simulink model "simple_arda_mpc_tune_me"  (R2021b)
settings: Solver=VariableStepAuto  StartTime=0  StopTime=10000  FixedStep=0.1  RelTol=1e-3
PreLoadFcn:
  | % Setup model parameters
  |                 % Sample time
  |                 %Ts = 0.1;
  |                 % Simulation stop time ("TimeOut")
  |                 %stop_time = 8000;
  |                 % Temperature
  |                 %T_init = 20 + 273.1755;
  |                % T_final = 294.1755;
  |               %  T_env = 20 + 273.15; %#ok<*NASGU>
  |              %   % Heater
  |                 %u_volts_heater_init = 0; % volts
  |                 % Pressure
  |                 %p_init = 101.325; % kPa
  |                 %p_env = 101.325; % kPa
  |                 % Relative humidity and steam
  |                 %phi_init = 0.4987;
  |                 %phi_final = 0.6;
  |                 %phi_env = 0.1;
  |                 %u_steam_init = 0;
  |                 %T_steam = 130 + 273.15;
  |                 % Volumetric flow rate
  |                 %u_volts_fan_init = 1;
  |                 %flow_init = 5.8e-3;
  |                 %flow_final = 0.18;
  |                 % Smooth ramp input parameters
  |                 %smooth_step_heater = make_smooth_step(0, T_init, T_final, Ts, stop_time, 'T_g');
  |                 %smooth_step_steam = make_smooth_step(0, phi_init, phi_final, Ts, stop_time, 'phi');
  |                 %smooth_step_fan = make_smooth_step(0, flow_init, flow_final, Ts, stop_time, 'flow');
  |                 % Parameters to vary for linearization
  |                 % Pipes
  |                 %pipe_length1 = 1; % meters
  |                 %pipe_length2 = 1;
  |                 %pipe_length3 = 1;
  |                 %pipe_cross_sectional_area1 = pi*(2*2.54/2)^2; % cm^2
  |                 %pipe_cross_sectional_area2 = pi*(2*2.54/2)^2;
  |                 %pipe_cross_sectional_area3 = pi*(2*2.54/2)^2;
  |                 %pipe_hydraulic_diameter1 = 2*2.54; %cm
  |                 %pipe_hydraulic_diameter2 = 2*2.54; %cm
  |                 %pipe_hydraulic_diameter3 = 2*2.54; %cm
  |                 % Thermal masses
  |                 %thermal_mass1 = 1; % kg
  |                 %thermal_mass2 = 1; % kg
  |                 %thermal_mass3 = 1; % kg
  |                 %thermal_mass4 = 1; % kg
  |                 %thermal_mass5 = 1; % kg
  |                 %specific_heat1 = 447; % J/(K*kg)
  |                 %specific_heat2 = 447; % J/(K*kg)
  |                 %specific_heat3 = 447; % J/(K*kg)
  |                 %specific_heat4 = 447; % J/(K*kg)
  |                 %specific_heat5 = 447; % J/(K*kg)
InitFcn:
  | load('bob.mat')
model workspace (MAT data in the model file):
  simple_arda_mpc_tune_me_sdosession = sldodialogs.data.SessionData
  simple_arda_mpc_tune_me_sdosession.Version = '3.0'
  simple_arda_mpc_tune_me_sdosession.Data.ModelName = 'simple_arda_mpc_tune_me'
  simple_arda_mpc_tune_me_sdosession.Data.ToolType = 'ResponseOptimization'
  simple_arda_mpc_tune_me_sdosession.Data.GUIOptions.NoPromptClose = 0
  simple_arda_mpc_tune_me_sdosession.Data.Workspace.LocalWorkspace.BlockReq = sldodialogs.databrowser.BlockRequirementData
  simple_arda_mpc_tune_me_sdosession.Data.Workspace.LocalWorkspace.BlockReq.Name = 'BlockReq'
  simple_arda_mpc_tune_me_sdosession.Data.Workspace.LocalWorkspace.BlockReq.Block = 'simple_arda_mpc_tune_me/check_T'
  simple_arda_mpc_tune_me_sdosession.Data.Workspace.LocalWorkspace.BlockReq_1 = sldodialogs.databrowser.BlockRequirementData
  simple_arda_mpc_tune_me_sdosession.Data.Workspace.LocalWorkspace.BlockReq_1.Name = 'BlockReq_1'
  simple_arda_mpc_tune_me_sdosession.Data.Workspace.LocalWorkspace.BlockReq_1.Block = 'simple_arda_mpc_tune_me/check_flow'
  simple_arda_mpc_tune_me_sdosession.Data.Workspace.LocalWorkspace.BlockReq_2 = sldodialogs.databrowser.BlockRequirementData
  simple_arda_mpc_tune_me_sdosession.Data.Workspace.LocalWorkspace.BlockReq_2.Name = 'BlockReq_2'
  simple_arda_mpc_tune_me_sdosession.Data.Workspace.LocalWorkspace.BlockReq_2.Block = 'simple_arda_mpc_tune_me/check_phi'
  simple_arda_mpc_tune_me_sdosession.Data.Workspace.LocalWorkspace.DesignVars(1) = param.Continuous
  simple_arda_mpc_tune_me_sdosession.Data.Workspace.LocalWorkspace.DesignVars(1).Minimum_ = 0
  simple_arda_mpc_tune_me_sdosession.Data.Workspace.LocalWorkspace.DesignVars(1).Maximum_ = 4
  simple_arda_mpc_tune_me_sdosession.Data.Workspace.LocalWorkspace.DesignVars(1).Scale_ = 2
  simple_arda_mpc_tune_me_sdosession.Data.Workspace.LocalWorkspace.DesignVars(1).Size_ = [1 1]
  simple_arda_mpc_tune_me_sdosession.Data.Workspace.LocalWorkspace.DesignVars(1).Value_ = 1.99942074063
  simple_arda_mpc_tune_me_sdosession.Data.Workspace.LocalWorkspace.DesignVars(1).pID = paramid.Variable
  simple_arda_mpc_tune_me_sdosession.Data.Workspace.LocalWorkspace.DesignVars(1).pID.Name = 'u1_wt'
  simple_arda_mpc_tune_me_sdosession.Data.Workspace.LocalWorkspace.DesignVars(2) = param.Continuous
  simple_arda_mpc_tune_me_sdosession.Data.Workspace.LocalWorkspace.DesignVars(2).Minimum_ = 3
  simple_arda_mpc_tune_me_sdosession.Data.Workspace.LocalWorkspace.DesignVars(2).Maximum_ = 6
  simple_arda_mpc_tune_me_sdosession.Data.Workspace.LocalWorkspace.DesignVars(2).Scale_ = 8
  simple_arda_mpc_tune_me_sdosession.Data.Workspace.LocalWorkspace.DesignVars(2).Size_ = [1 1]
  simple_arda_mpc_tune_me_sdosession.Data.Workspace.LocalWorkspace.DesignVars(2).Value_ = 4.47918835767
  simple_arda_mpc_tune_me_sdosession.Data.Workspace.LocalWorkspace.DesignVars(2).pID = paramid.Variable
  simple_arda_mpc_tune_me_sdosession.Data.Workspace.LocalWorkspace.DesignVars(2).pID.Name = 'u2_wt'
  simple_arda_mpc_tune_me_sdosession.Data.Workspace.LocalWorkspace.DesignVars(3) = param.Continuous
  simple_arda_mpc_tune_me_sdosession.Data.Workspace.LocalWorkspace.DesignVars(3).Minimum_ = 6
  simple_arda_mpc_tune_me_sdosession.Data.Workspace.LocalWorkspace.DesignVars(3).Maximum_ = 10
  simple_arda_mpc_tune_me_sdosession.Data.Workspace.LocalWorkspace.DesignVars(3).Scale_ = 8
  simple_arda_mpc_tune_me_sdosession.Data.Workspace.LocalWorkspace.DesignVars(3).Size_ = [1 1]
  simple_arda_mpc_tune_me_sdosession.Data.Workspace.LocalWorkspace.DesignVars(3).Value_ = 6
  simple_arda_mpc_tune_me_sdosession.Data.Workspace.LocalWorkspace.DesignVars(3).pID = paramid.Variable
  simple_arda_mpc_tune_me_sdosession.Data.Workspace.LocalWorkspace.DesignVars(3).pID.Name = 'u3_wt'
  simple_arda_mpc_tune_me_sdosession.Data.Workspace.LocalWorkspace.DesignVars(4) = param.Continuous
  simple_arda_mpc_tune_me_sdosession.Data.Workspace.LocalWorkspace.DesignVars(4).Minimum_ = 850
  simple_arda_mpc_tune_me_sdosession.Data.Workspace.LocalWorkspace.DesignVars(4).Maximum_ = 1050
  simple_arda_mpc_tune_me_sdosession.Data.Workspace.LocalWorkspace.DesignVars(4).Scale_ = 1024
  simple_arda_mpc_tune_me_sdosession.Data.Workspace.LocalWorkspace.DesignVars(4).Size_ = [1 1]
  simple_arda_mpc_tune_me_sdosession.Data.Workspace.LocalWorkspace.DesignVars(4).Value_ = 1050
  simple_arda_mpc_tune_me_sdosession.Data.Workspace.LocalWorkspace.DesignVars(4).pID = paramid.Variable
  simple_arda_mpc_tune_me_sdosession.Data.Workspace.LocalWorkspace.DesignVars(4).pID.Name = 'y1_wt'
  simple_arda_mpc_tune_me_sdosession.Data.Workspace.LocalWorkspace.DesignVars(5) = param.Continuous
  simple_arda_mpc_tune_me_sdosession.Data.Workspace.LocalWorkspace.DesignVars(5).Minimum_ = 38
  simple_arda_mpc_tune_me_sdosession.Data.Workspace.LocalWorkspace.DesignVars(5).Maximum_ = 46
  simple_arda_mpc_tune_me_sdosession.Data.Workspace.LocalWorkspace.DesignVars(5).Scale_ = 64
  simple_arda_mpc_tune_me_sdosession.Data.Workspace.LocalWorkspace.DesignVars(5).Size_ = [1 1]
  simple_arda_mpc_tune_me_sdosession.Data.Workspace.LocalWorkspace.DesignVars(5).Value_ = 46
  simple_arda_mpc_tune_me_sdosession.Data.Workspace.LocalWorkspace.DesignVars(5).pID = paramid.Variable
  simple_arda_mpc_tune_me_sdosession.Data.Workspace.LocalWorkspace.DesignVars(5).pID.Name = 'y2_wt'
  simple_arda_mpc_tune_me_sdosession.Data.Workspace.LocalWorkspace.DesignVars(6) = param.Continuous
  simple_arda_mpc_tune_me_sdosession.Data.Workspace.LocalWorkspace.DesignVars(6).Minimum_ = 200
  simple_arda_mpc_tune_me_sdosession.Data.Workspace.LocalWorkspace.DesignVars(6).Maximum_ = 250
  simple_arda_mpc_tune_me_sdosession.Data.Workspace.LocalWorkspace.DesignVars(6).Scale_ = 256
  simple_arda_mpc_tune_me_sdosession.Data.Workspace.LocalWorkspace.DesignVars(6).Size_ = [1 1]
  simple_arda_mpc_tune_me_sdosession.Data.Workspace.LocalWorkspace.DesignVars(6).Value_ = 200
  simple_arda_mpc_tune_me_sdosession.Data.Workspace.LocalWorkspace.DesignVars(6).pID = paramid.Variable
  simple_arda_mpc_tune_me_sdosession.Data.Workspace.LocalWorkspace.DesignVars(6).pID.Name = 'y3_wt'
  simple_arda_mpc_tune_me_sdosession.Data.Workspace.LocalWorkspace.DesignVars(7) = param.Continuous
  simple_arda_mpc_tune_me_sdosession.Data.Workspace.LocalWorkspace.DesignVars(7).Minimum_ = 4000
  simple_arda_mpc_tune_me_sdosession.Data.Workspace.LocalWorkspace.DesignVars(7).Maximum_ = 6000
  simple_arda_mpc_tune_me_sdosession.Data.Workspace.LocalWorkspace.DesignVars(7).Scale_ = 8192
  simple_arda_mpc_tune_me_sdosession.Data.Workspace.LocalWorkspace.DesignVars(7).Size_ = [1 1]
  simple_arda_mpc_tune_me_sdosession.Data.Workspace.LocalWorkspace.DesignVars(7).Value_ = 5000
  simple_arda_mpc_tune_me_sdosession.Data.Workspace.LocalWorkspace.DesignVars(7).pID = paramid.Variable
  simple_arda_mpc_tune_me_sdosession.Data.Workspace.LocalWorkspace.DesignVars(7).pID.Name = 'u1p_wt'
  simple_arda_mpc_tune_me_sdosession.Data.Workspace.LocalWorkspace.DesignVars(8) = param.Continuous
  simple_arda_mpc_tune_me_sdosession.Data.Workspace.LocalWorkspace.DesignVars(8).Minimum_ = 2000
  simple_arda_mpc_tune_me_sdosession.Data.Workspace.LocalWorkspace.DesignVars(8).Maximum_ = 4000
  simple_arda_mpc_tune_me_sdosession.Data.Workspace.LocalWorkspace.DesignVars(8).Scale_ = 4096
  simple_arda_mpc_tune_me_sdosession.Data.Workspace.LocalWorkspace.DesignVars(8).Size_ = [1 1]
  simple_arda_mpc_tune_me_sdosession.Data.Workspace.LocalWorkspace.DesignVars(8).Value_ = 3000
  simple_arda_mpc_tune_me_sdosession.Data.Workspace.LocalWorkspace.DesignVars(8).pID = paramid.Variable
  simple_arda_mpc_tune_me_sdosession.Data.Workspace.LocalWorkspace.DesignVars(8).pID.Name = 'u2p_wt'
  simple_arda_mpc_tune_me_sdosession.Data.Workspace.LocalWorkspace.DesignVars(9) = param.Continuous
  simple_arda_mpc_tune_me_sdosession.Data.Workspace.LocalWorkspace.DesignVars(9).Minimum_ = 1000
  simple_arda_mpc_tune_me_sdosession.Data.Workspace.LocalWorkspace.DesignVars(9).Maximum_ = 3000
  simple_arda_mpc_tune_me_sdosession.Data.Workspace.LocalWorkspace.DesignVars(9).Scale_ = 2048
  simple_arda_mpc_tune_me_sdosession.Data.Workspace.LocalWorkspace.DesignVars(9).Size_ = [1 1]
  simple_arda_mpc_tune_me_sdosession.Data.Workspace.LocalWorkspace.DesignVars(9).Value_ = 2000
  simple_arda_mpc_tune_me_sdosession.Data.Workspace.LocalWorkspace.DesignVars(9).pID = paramid.Variable
  simple_arda_mpc_tune_me_sdosession.Data.Workspace.LocalWorkspace.DesignVars(9).pID.Name = 'u3p_wt'
  simple_arda_mpc_tune_me_sdosession.Data.Workspace.LocalWorkspace.DesignVars(10) = param.Continuous
  simple_arda_mpc_tune_me_sdosession.Data.Workspace.LocalWorkspace.DesignVars(10).Minimum_ = 1
  simple_arda_mpc_tune_me_sdosession.Data.Workspace.LocalWorkspace.DesignVars(10).Maximum_ = 4
  simple_arda_mpc_tune_me_sdosession.Data.Workspace.LocalWorkspace.DesignVars(10).Scale_ = 8
  simple_arda_mpc_tune_me_sdosession.Data.Workspace.LocalWorkspace.DesignVars(10).Size_ = [1 1]
  simple_arda_mpc_tune_me_sdosession.Data.Workspace.LocalWorkspace.DesignVars(10).Value_ = 5
  simple_arda_mpc_tune_me_sdosession.Data.Workspace.LocalWorkspace.DesignVars(10).pID = paramid.Variable
  simple_arda_mpc_tune_me_sdosession.Data.Workspace.LocalWorkspace.DesignVars(10).pID.Name = 'control_horizon'
  simple_arda_mpc_tune_me_sdosession.Data.Workspace.LocalWorkspace.DesignVars(11) = param.Continuous
  simple_arda_mpc_tune_me_sdosession.Data.Workspace.LocalWorkspace.DesignVars(11).Minimum_ = 5
  simple_arda_mpc_tune_me_sdosession.Data.Workspace.LocalWorkspace.DesignVars(11).Maximum_ = 10
  simple_arda_mpc_tune_me_sdosession.Data.Workspace.LocalWorkspace.DesignVars(11).Scale_ = 16
  simple_arda_mpc_tune_me_sdosession.Data.Workspace.LocalWorkspace.DesignVars(11).Size_ = [1 1]
  simple_arda_mpc_tune_me_sdosession.Data.Workspace.LocalWorkspace.DesignVars(11).Value_ = 10
  simple_arda_mpc_tune_me_sdosession.Data.Workspace.LocalWorkspace.DesignVars(11).pID = paramid.Variable
  simple_arda_mpc_tune_me_sdosession.Data.Workspace.LocalWorkspace.DesignVars(11).pID.Name = 'prediction_horizon'
  simple_arda_mpc_tune_me_sdosession.Data.Workspace.LocalWorkspace.ReqValues(1).Name = 'simple_arda_mpc_tune_me/check_T (Upper)'
  simple_arda_mpc_tune_me_sdosession.Data.Workspace.LocalWorkspace.ReqValues(1).Type = '<='
  simple_arda_mpc_tune_me_sdosession.Data.Workspace.LocalWorkspace.ReqValues(1).Value = [-0.0594490574926; -0.054838686924; -0.0546633029945; -0.000573871237779; 0.0439457003428; 0.0538224147144; 0.0538106463197; 436.002710593]
  simple_arda_mpc_tune_me_sdosession.Data.Workspace.LocalWorkspace.ReqValues(1).DisplayValue = [-0.0594490574926; -0.054838686924; -0.0546633029945; -0.000573871237779; 0.0439457003428; 0.0538224147144; 0.0538106463197; 436.002710593]
  simple_arda_mpc_tune_me_sdosession.Data.Workspace.LocalWorkspace.ReqValues(2).Name = 'simple_arda_mpc_tune_me/check_flow (Upper)'
  simple_arda_mpc_tune_me_sdosession.Data.Workspace.LocalWorkspace.ReqValues(2).Type = '<='
  simple_arda_mpc_tune_me_sdosession.Data.Workspace.LocalWorkspace.ReqValues(2).Value = [-0.954656561585; -0.967742763883; -0.947580933078; -1.05584644778; 0.959275239402; 0.975371838836; 0.991305602274; 924.477313265]
  simple_arda_mpc_tune_me_sdosession.Data.Workspace.LocalWorkspace.ReqValues(2).DisplayValue = [-0.954656561585; -0.967742763883; -0.947580933078; -1.05584644778; 0.959275239402; 0.975371838836; 0.991305602274; 924.477313265]
  simple_arda_mpc_tune_me_sdosession.Data.Workspace.LocalWorkspace.ReqValues(3).Name = 'simple_arda_mpc_tune_me/check_phi (Upper)'
  simple_arda_mpc_tune_me_sdosession.Data.Workspace.LocalWorkspace.ReqValues(3).Type = '<='
  simple_arda_mpc_tune_me_sdosession.Data.Workspace.LocalWorkspace.ReqValues(3).Value = [-0.400637667521; 0.0893932441366]
  simple_arda_mpc_tune_me_sdosession.Data.Workspace.LocalWorkspace.ReqValues(3).DisplayValue = [-0.400637667521; 0.0893932441366]
  simple_arda_mpc_tune_me_sdosession.Data.Workspace.LocalWorkspace.ReqValues(4).Name = 'simple_arda_mpc_tune_me/check_phi (Lower)'
  simple_arda_mpc_tune_me_sdosession.Data.Workspace.LocalWorkspace.ReqValues(4).Type = '>='
  simple_arda_mpc_tune_me_sdosession.Data.Workspace.LocalWorkspace.ReqValues(4).Value = [-0.599166284275; -0.330396343818]
  simple_arda_mpc_tune_me_sdosession.Data.Workspace.LocalWorkspace.ReqValues(4).DisplayValue = [0.599166284275; 0.330396343818]
  simple_arda_mpc_tune_me_sdosession.Data.Workspace.HiddenWorkspace = []
  simple_arda_mpc_tune_me_sdosession.Data.ToolData.PlotManager.Plots(1).Class = 'block'
  simple_arda_mpc_tune_me_sdosession.Data.ToolData.PlotManager.Plots(1).Sources = {'simple_arda_mpc_tune_me/check_T'}
  simple_arda_mpc_tune_me_sdosession.Data.ToolData.PlotManager.Plots(2).Class = 'block'
  simple_arda_mpc_tune_me_sdosession.Data.ToolData.PlotManager.Plots(2).Sources = {'simple_arda_mpc_tune_me/check_flow'}
  simple_arda_mpc_tune_me_sdosession.Data.ToolData.PlotManager.Plots(3).Class = 'block'
  simple_arda_mpc_tune_me_sdosession.Data.ToolData.PlotManager.Plots(3).Sources = {'simple_arda_mpc_tune_me/check_phi'}
  simple_arda_mpc_tune_me_sdosession.Data.ToolData.PlotManager.Plots(4).Class = 'sldoplots.IterPlot'
  simple_arda_mpc_tune_me_sdosession.Data.ToolData.PlotManager.Plots(4).Sources = {'DesignVars'}
  simple_arda_mpc_tune_me_sdosession.Data.ToolData.PlotManager.Tiling : java.lang.String (value not decoded)
  simple_arda_mpc_tune_me_sdosession.Data.ToolData.DialogManager = []
  simple_arda_mpc_tune_me_sdosession.Data.ToolData.ResponseOptimization.Options = sdo.OptimizeOptions
  simple_arda_mpc_tune_me_sdosession.Data.ToolData.ResponseOptimization.Options.Restarts = 2
  simple_arda_mpc_tune_me_sdosession.Data.ToolData.ResponseOptimization.Options.UseParallel = 1
  simple_arda_mpc_tune_me_sdosession.Data.ToolData.ResponseOptimization.Options.ParallelFileDependencies = {'C:/Users/dmeissner/stuff/arda/work/integration/bob.mat'; 'C:/Users/dmeissner/stuff/arda/work/integration/data_dictionary1.sldd'; 'C:/Users/dmeissner/stuff/arda/work/integration/plant.slx'; 'C:/Users/dmeissner/stuff/arda/work/integration/simple_arda_mpc_tune_me.slx'; 'C:/Users/dmeissner/stuff/arda/work/integration/simple_arda_mpc_tune_me.slxc'}
  simple_arda_mpc_tune_me_sdosession.Data.ToolData.ResponseOptimization.Options.OptimizedModel = 'simple_arda_mpc_tune_me'
  simple_arda_mpc_tune_me_sdosession.Data.ToolData.ResponseOptimization.Options.Version = 2
  simple_arda_mpc_tune_me_sdosession.Data.ToolData.ResponseOptimization.GUIOptions.ModelTimeOut = 15000
  simple_arda_mpc_tune_me_sdosession.Data.ToolData.ResponseOptimization.GUIOptions.ComputeOperatingPoint = 0
  simple_arda_mpc_tune_me_sdosession.Data.ToolData.ResponseOptimization.GUIOptions.ShowProgress = 1
  simple_arda_mpc_tune_me_sdosession.Data.ToolData.ResponseOptimization.GUIOptions.ShowParamTrajectory = 1
  simple_arda_mpc_tune_me_sdosession.Data.ToolData.ResponseOptimization.GUIOptions.UpdatePlots = 0
  simple_arda_mpc_tune_me_sdosession.Data.ToolData.ResponseOptimization.GUIOptions.UpdateModel = 1
  simple_arda_mpc_tune_me_sdosession.Data.ToolData.ResponseOptimization.GUIOptions.UpdateDesign = 'overwrite'
  simple_arda_mpc_tune_me_sdosession.Data.ToolData.ResponseOptimization.GUIOptions.SaveReport = 0
  simple_arda_mpc_tune_me_sdosession.Data.ToolData.ResponseOptimization.GUIOptions.SaveRequirementValue = 1
  simple_arda_mpc_tune_me_sdosession.Data.ToolData.ResponseOptimization.LinOptions = linearize.LinearizeOptions
  simple_arda_mpc_tune_me_sdosession.Data.ToolData.ResponseOptimization.RequirementOperatingPointSetup = []
  simple_arda_mpc_tune_me_sdosession.Data.ToolData.ResponseOptimization.LocalRequirements = struct([])
  simple_arda_mpc_tune_me_sdosession.Data.ToolData.ResponseOptimization.BlockRequirements(1).Block = 'simple_arda_mpc_tune_me/check_T'
  simple_arda_mpc_tune_me_sdosession.Data.ToolData.ResponseOptimization.BlockRequirements(1).Selected = 1
  simple_arda_mpc_tune_me_sdosession.Data.ToolData.ResponseOptimization.BlockRequirements(1).hReq = sdo.requirements.StepResponseEnvelope
  simple_arda_mpc_tune_me_sdosession.Data.ToolData.ResponseOptimization.BlockRequirements(1).hReq.sdo.requirements.Requirement.Data_ : srorequirement.steprespdata (value not decoded)
  simple_arda_mpc_tune_me_sdosession.Data.ToolData.ResponseOptimization.BlockRequirements(1).hReq.sdo.requirements.Requirement.Check_ = sdo.requirements.PiecewiseLinearCheck
  simple_arda_mpc_tune_me_sdosession.Data.ToolData.ResponseOptimization.BlockRequirements(1).hReq.sdo.requirements.Requirement.Check_.Orientation = 'horizontal'
  simple_arda_mpc_tune_me_sdosession.Data.ToolData.ResponseOptimization.BlockRequirements(1).hReq.sdo.requirements.Requirement.Check_.XScale = 'linear'
  simple_arda_mpc_tune_me_sdosession.Data.ToolData.ResponseOptimization.BlockRequirements(2).Block = 'simple_arda_mpc_tune_me/check_flow'
  simple_arda_mpc_tune_me_sdosession.Data.ToolData.ResponseOptimization.BlockRequirements(2).Selected = 1
  simple_arda_mpc_tune_me_sdosession.Data.ToolData.ResponseOptimization.BlockRequirements(2).hReq = sdo.requirements.StepResponseEnvelope
  simple_arda_mpc_tune_me_sdosession.Data.ToolData.ResponseOptimization.BlockRequirements(2).hReq.sdo.requirements.Requirement.Data_ : srorequirement.steprespdata (value not decoded)
  simple_arda_mpc_tune_me_sdosession.Data.ToolData.ResponseOptimization.BlockRequirements(2).hReq.sdo.requirements.Requirement.Check_ = sdo.requirements.PiecewiseLinearCheck
  simple_arda_mpc_tune_me_sdosession.Data.ToolData.ResponseOptimization.BlockRequirements(2).hReq.sdo.requirements.Requirement.Check_.Orientation = 'horizontal'
  simple_arda_mpc_tune_me_sdosession.Data.ToolData.ResponseOptimization.BlockRequirements(2).hReq.sdo.requirements.Requirement.Check_.XScale = 'linear'
  simple_arda_mpc_tune_me_sdosession.Data.ToolData.ResponseOptimization.BlockRequirements(3).Block = 'simple_arda_mpc_tune_me/check_phi'
  simple_arda_mpc_tune_me_sdosession.Data.ToolData.ResponseOptimization.BlockRequirements(3).Selected = 1
  simple_arda_mpc_tune_me_sdosession.Data.ToolData.ResponseOptimization.BlockRequirements(3).hReq(1) = sdo.requirements.SignalBound
  simple_arda_mpc_tune_me_sdosession.Data.ToolData.ResponseOptimization.BlockRequirements(3).hReq(1).sdo.requirements.Requirement.Data_ : srorequirement.piecewisedata (value not decoded)
  simple_arda_mpc_tune_me_sdosession.Data.ToolData.ResponseOptimization.BlockRequirements(3).hReq(1).sdo.requirements.Requirement.Check_ = sdo.requirements.PiecewiseLinearCheck
  simple_arda_mpc_tune_me_sdosession.Data.ToolData.ResponseOptimization.BlockRequirements(3).hReq(1).sdo.requirements.Requirement.Check_.Orientation = 'horizontal'
  simple_arda_mpc_tune_me_sdosession.Data.ToolData.ResponseOptimization.BlockRequirements(3).hReq(1).sdo.requirements.Requirement.Check_.XScale = 'linear'
  simple_arda_mpc_tune_me_sdosession.Data.ToolData.ResponseOptimization.BlockRequirements(3).hReq(2) = sdo.requirements.SignalBound
  simple_arda_mpc_tune_me_sdosession.Data.ToolData.ResponseOptimization.BlockRequirements(3).hReq(2).sdo.requirements.Requirement.Data_ : srorequirement.piecewisedata (value not decoded)
  simple_arda_mpc_tune_me_sdosession.Data.ToolData.ResponseOptimization.BlockRequirements(3).hReq(2).sdo.requirements.Requirement.Check_ = sdo.requirements.PiecewiseLinearCheck
  simple_arda_mpc_tune_me_sdosession.Data.ToolData.ResponseOptimization.BlockRequirements(3).hReq(2).sdo.requirements.Requirement.Check_.Orientation = 'horizontal'
  simple_arda_mpc_tune_me_sdosession.Data.ToolData.ResponseOptimization.BlockRequirements(3).hReq(2).sdo.requirements.Requirement.Check_.XScale = 'linear'
  simple_arda_mpc_tune_me_sdosession.Data.ToolData.ResponseOptimization.LocalExperiments = struct([])
  simple_arda_mpc_tune_me_sdosession.Data.ToolData.ResponseOptimization.Cost.Type = 'SSE'
  simple_arda_mpc_tune_me_sdosession.Data.ToolData.ResponseOptimization.Cost.Robust = 'off'
  simple_arda_mpc_tune_me_sdosession.Data.ToolData.ResponseOptimization.DesignVariables = 'DesignVars'
  simple_arda_mpc_tune_me_sdosession.Data.ToolData.ResponseOptimization.UncertainVariables = ''
  simple_arda_mpc_tune_me_sdosession.Data.ToolData.ResponseOptimization.DataToPlot = 'DesignVars'
values from neighbouring files (symbols this model uses):
  control_horizon = 1.0    [data_dictionary1.sldd]
  ecr_wt = 100000.0    [data_dictionary1.sldd]
  flow_init = 0.0    [data_dictionary1.sldd]
  phi = x(9)    [odefun.m]
  phi_init = 0.6    [data_dictionary1.sldd]
  prediction_horizon = 10.0    [data_dictionary1.sldd]
  T_init = 293.15    [data_dictionary1.sldd]
  u1_wt = 1.9994207406305169    [data_dictionary1.sldd]
  u1p_wt = 5000.0    [data_dictionary1.sldd]
  u2_wt = 4.4791883576650164    [data_dictionary1.sldd]
  u2p_wt = 200000.0    [data_dictionary1.sldd]
  u3_wt = 6.0    [data_dictionary1.sldd]
  u3p_wt = 2000.0    [data_dictionary1.sldd]
  y1_wt = 1050.0    [data_dictionary1.sldd]
  y2_wt = 46.0    [data_dictionary1.sldd]
  y3_wt = 200.0    [data_dictionary1.sldd]
libraries: simulink x3, checkpacklib x3, mpclib x1
settings Model: DataDictionary=data_dictionary1.sldd  Creator=dmeissner  LastModifiedBy=dmeissner
settings SolverCC: ZeroCrossAlgorithm=Adaptive
settings DataIOCC: DSMLogging=off  ReturnWorkspaceOutputsName=SDOSimTest_Log
settings DebuggingCC: ModelReferenceIOMsg=warning  ModelReferenceVersionMismatchMessage=warning  ModelReferenceIOMismatchMessage=warning  ModelReferenceNoExplicitFinalValueMsg=warning

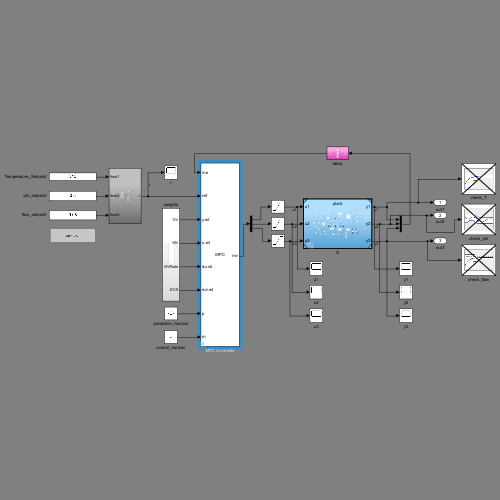
[thumbnail: Simulink's stored preview of the top-level diagram]
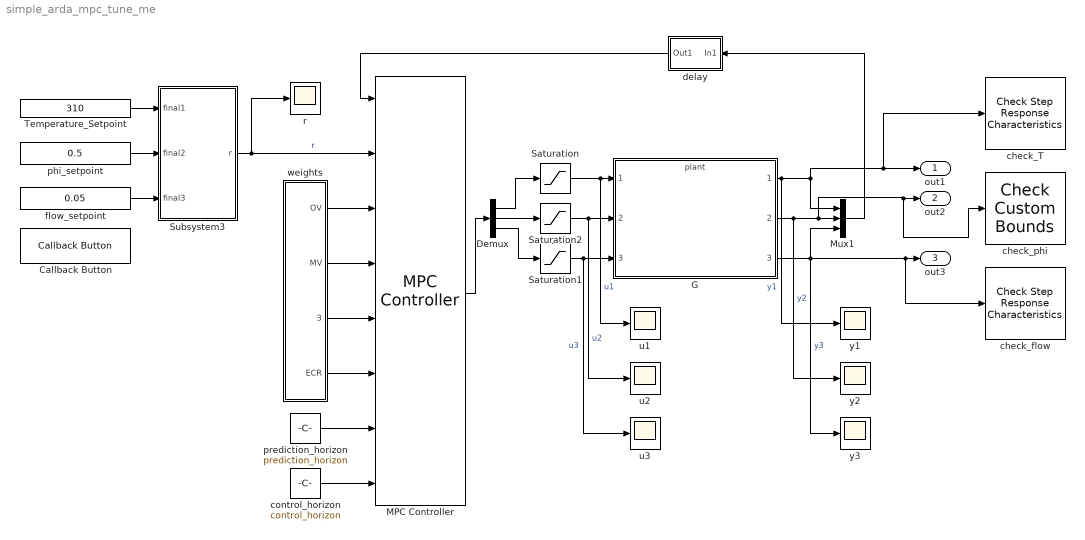
== system simple_arda_mpc_tune_me ==
  Callback Button : CallbackButton  ButtonText=phi + 0.01
      settings: ClickFcn=|
      | phi_setpoint = str2num(get_param('simple_arda_mpc_tune_me/phi_setpoint',"Value"))
      | phi_setpoint = phi_setpoint + 0.01
      | set_param('simple_arda_mpc_tune_me/phi_setpoint',"Value", num2str(phi_setpoint))
  Demux : Demux  Outputs=3
  G : ModelReference  ModelNameDialog=plant.slx  SimulationMode=Normal  ModelReferenceVersion=1.184
  MPC Controller : mpclib/MPC Controller  SCDEnableBlockLinearizationSpecification=on  mpcobj=bob.controller.mpc1  x0=bob.controller.mpc1_initial_state  is_multiple=0  enable_value=0  return_u0=off  updateMPCinCallerWorkspace=on  md_inport=off  mv_inport=off  uref_inport=off  return_cost=off  return_mvseq=off  return_qpstatus=off  return_xseq=off  return_state=off  return_ovseq=off  state_inport=off  umin_inport=off  umax_inport=off  ymin_inport=off  ymax_inport=off  cc_inport=off  ywt_inport=on  uwt_inport=on  duwt_inport=on  rhoeps_inport=on  pm_inport=on  MaximumP=10  HorizonChoice=VariableHorizon  n_ts=0.1  n_p=10  n_mv=3  n_md=0  n_ud=0  n_mo=3  n_uo=0  BlockDataType=double  SampleTimeInherited=off  switch_inport=off
  Mux1 : Mux  Inputs=3
  Saturation : Saturate  UpperLimit=460  LowerLimit=0
  Saturation1 : Saturate  UpperLimit=460  LowerLimit=0
  Saturation2 : Saturate  UpperLimit=0.06  LowerLimit=0
  Subsystem3 : Subsystem
  Temperature_Setpoint : Constant  Value=310
  check_T : checkpacklib/Check Step Response  Characteristics  InstantiateOnLoad=on  enabled=off  stopWhenAssertionFail=off  export=off  ViewDlgPos=[113 42 510 390]  OpenViewOnLoad=off  LaunchViewOnOpen=off  TimeUnits=seconds  EnableStepResponseBound=on  InitialValue=293.15  FinalValue=310  StepTime=1  RiseTime=3500  PercentRise=80  SettlingTime=4000  PercentSettling=1  PercentOvershoot=10  PercentUndershoot=1
      settings: SourceProductBaseCode=CT,ID,MT,SO
  check_flow : checkpacklib/Check Step Response  Characteristics  InstantiateOnLoad=on  enabled=off  stopWhenAssertionFail=off  export=off  ViewDlgPos=[100 200 510 390]  OpenViewOnLoad=off  LaunchViewOnOpen=off  TimeUnits=seconds  EnableStepResponseBound=on  InitialValue=0  FinalValue=0.18  StepTime=1  RiseTime=20  PercentRise=80  SettlingTime=30  PercentSettling=1  PercentOvershoot=10  PercentUndershoot=1
      settings: SourceProductBaseCode=CT,ID,MT,SO
  check_phi : checkpacklib/Check Custom Bounds  InstantiateOnLoad=on  enabled=off  stopWhenAssertionFail=off  export=off  ViewDlgPos=[]  OpenViewOnLoad=off  LaunchViewOnOpen=off  TimeUnits=seconds  EnableUpperBound=on  UpperBoundTimes=[0 3500; 3500 10000]  UpperBoundAmplitudes=[1 1; 0.55 0.55];  EnableLowerBound=on  LowerBoundTimes=[0 3500; 3500 10000]  LowerBoundAmplitudes=[0 0; 0.45 0.45]
      settings: SourceProductBaseCode=CT,ID,MT,SO
  control_horizon : Constant  Value=control_horizon
  delay : Subsystem
  flow_setpoint : Constant  Value=0.05
  phi_setpoint : Constant  Value=0.5
  prediction_horizon : Constant  Value=prediction_horizon
  r : Scope
  u1 : Scope
  u2 : Scope
  u3 : Scope
  weights : Subsystem
  y1 : Scope
  y2 : Scope
  y3 : Scope
  out1 : Outport
  out2 : Outport  Port=2
  out3 : Outport  Port=3
  wires:
  G/2 -> check_phi/1, out2/1, Mux1/2, y2/1  "y2"
  G/1 -> Mux1/1, check_T/1, out1/1, y1/1  "y1"
  G/3 -> y3/1, check_flow/1, out3/1, Mux1/3  "y3"
  Saturation/1 -> u1/1, G/1  "u1"
  Saturation2/1 -> u2/1, G/2  "u2"
  Saturation1/1 -> u3/1, G/3  "u3"
  Mux1/1 -> delay/1(In1)
  delay/1(Out1) -> MPC Controller/1
  Subsystem3/1(r) -> r/1, MPC Controller/2  "r"
  Demux/1 -> Saturation/1
  Demux/2 -> Saturation2/1
  Demux/3 -> Saturation1/1
  MPC Controller/1 -> Demux/1
  Temperature_Setpoint/1 -> Subsystem3/1(final1)
  phi_setpoint/1 -> Subsystem3/2(final2)
  flow_setpoint/1 -> Subsystem3/3(final3)
  weights/1(OV) -> MPC Controller/3
  weights/2(MV) -> MPC Controller/4
  weights/3(MVRate) -> MPC Controller/5
  weights/4(ECR) -> MPC Controller/6
  prediction_horizon/1 -> MPC Controller/7
  control_horizon/1 -> MPC Controller/8

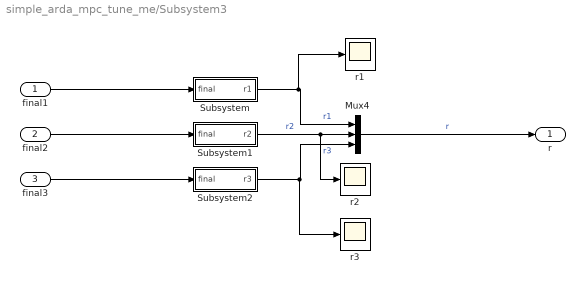
== system simple_arda_mpc_tune_me/Subsystem3 ==
  final1 : Inport
  final2 : Inport  Port=2
  final3 : Inport  Port=3
  Mux4 : Mux  Inputs=3
  Subsystem : Subsystem
  Subsystem1 : Subsystem
  Subsystem2 : Subsystem
  r1 : Scope
  r2 : Scope
  r3 : Scope
  r : Outport
  wires:
  final2/1 -> Subsystem1/1(final)
  Subsystem1/1(r2) -> r2/1, Mux4/2  "r2"
  Subsystem2/1(r3) -> r3/1, Mux4/3  "r3"
  Subsystem/1(r1) -> r1/1, Mux4/1  "r1"
  final1/1 -> Subsystem/1(final)
  final3/1 -> Subsystem2/1(final)
  Mux4/1 -> r/1  "r"

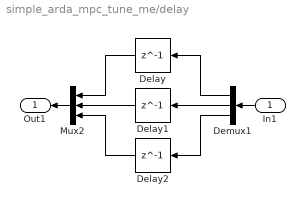
== system simple_arda_mpc_tune_me/delay ==
  In1 : Inport
  Delay : Delay  DelayLength=1
  Delay1 : Delay  DelayLength=1
  Delay2 : Delay  DelayLength=1
  Demux1 : Demux  Outputs=3
  Mux2 : Mux  Inputs=3
  Out1 : Outport
  wires:
  Mux2/1 -> Out1/1
  Demux1/2 -> Delay1/1
  In1/1 -> Demux1/1
  Delay1/1 -> Mux2/2
  Demux1/3 -> Delay2/1
  Delay/1 -> Mux2/1
  Demux1/1 -> Delay/1
  Delay2/1 -> Mux2/3

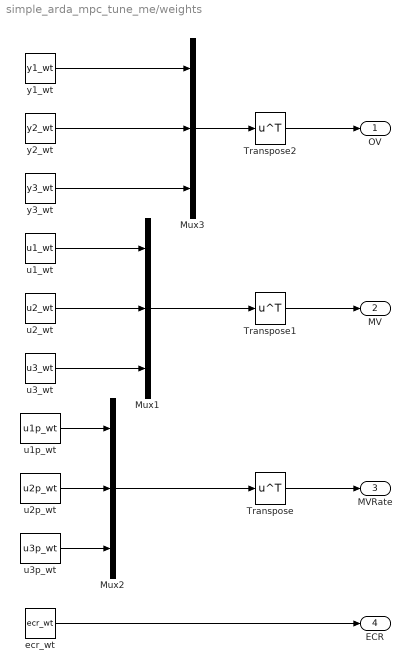
== system simple_arda_mpc_tune_me/weights ==
  Mux1 : Mux  Inputs=3
  Mux2 : Mux  Inputs=3
  Mux3 : Mux  Inputs=3
  Transpose : Math  Operator=transpose  SaturateOnIntegerOverflow=on
  Transpose1 : Math  Operator=transpose  SaturateOnIntegerOverflow=on
  Transpose2 : Math  Operator=transpose  SaturateOnIntegerOverflow=on
  ecr_wt : Constant  Value=ecr_wt
  u1_wt : Constant  Value=u1_wt
  u1p_wt : Constant  Value=u1p_wt
  u2_wt : Constant  Value=u2_wt
  u2p_wt : Constant  Value=u2p_wt
  u3_wt : Constant  Value=u3_wt
  u3p_wt : Constant  Value=u3p_wt
  y1_wt : Constant  Value=y1_wt
  y2_wt : Constant  Value=y2_wt
  y3_wt : Constant  Value=y3_wt
  OV : Outport
  MV : Outport  Port=2
  MVRate : Outport  Port=3
  ECR : Outport  Port=4
  wires:
  ecr_wt/1 -> ECR/1
  Transpose2/1 -> OV/1
  Transpose1/1 -> MV/1
  Transpose/1 -> MVRate/1
  y1_wt/1 -> Mux3/1
  y2_wt/1 -> Mux3/2
  y3_wt/1 -> Mux3/3
  u1_wt/1 -> Mux1/1
  u2_wt/1 -> Mux1/2
  u3_wt/1 -> Mux1/3
  u1p_wt/1 -> Mux2/1
  u2p_wt/1 -> Mux2/2
  u3p_wt/1 -> Mux2/3
  Mux3/1 -> Transpose2/1
  Mux1/1 -> Transpose1/1
  Mux2/1 -> Transpose/1

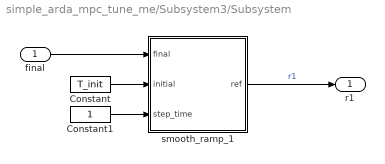
== system simple_arda_mpc_tune_me/Subsystem3/Subsystem ==
  final : Inport
  Constant : Constant  Value=T_init
  Constant1 : Constant
  smooth_ramp_1 : Subsystem
  r1 : Outport
  wires:
  Constant1/1 -> smooth_ramp_1/3(step_time)
  smooth_ramp_1/1(ref) -> r1/1  "r1"
  Constant/1 -> smooth_ramp_1/2(initial)
  final/1 -> smooth_ramp_1/1(final)

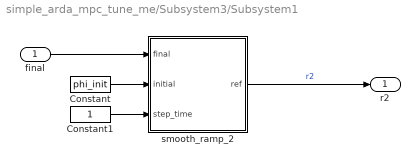
== system simple_arda_mpc_tune_me/Subsystem3/Subsystem1 ==
  final : Inport
  Constant : Constant  Value=phi_init
  Constant1 : Constant
  smooth_ramp_2 : Subsystem
  r2 : Outport
  wires:
  final/1 -> smooth_ramp_2/1(final)
  Constant/1 -> smooth_ramp_2/2(initial)
  smooth_ramp_2/1(ref) -> r2/1  "r2"
  Constant1/1 -> smooth_ramp_2/3(step_time)

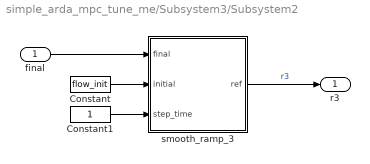
== system simple_arda_mpc_tune_me/Subsystem3/Subsystem2 ==
  final : Inport
  Constant : Constant  Value=flow_init
  Constant1 : Constant
  smooth_ramp_3 : Subsystem
  r3 : Outport
  wires:
  Constant1/1 -> smooth_ramp_3/3(step_time)
  smooth_ramp_3/1(ref) -> r3/1  "r3"
  Constant/1 -> smooth_ramp_3/2(initial)
  final/1 -> smooth_ramp_3/1(final)

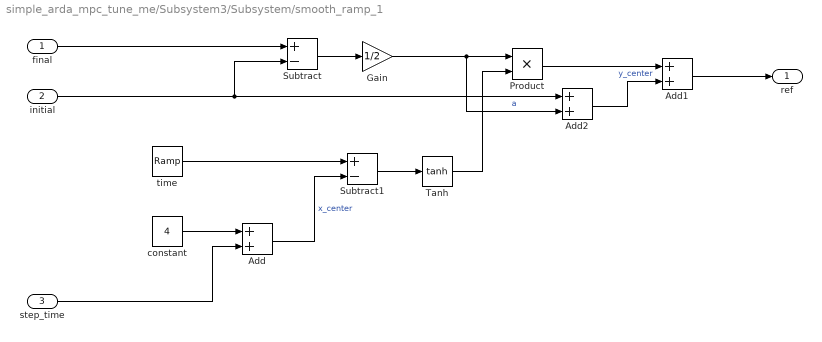
== system simple_arda_mpc_tune_me/Subsystem3/Subsystem/smooth_ramp_1 ==
  final : Inport
  initial : Inport  Port=2
  step_time : Inport  Port=3
  Add : Sum
  Add1 : Sum
  Add2 : Sum
  Gain : Gain  Gain=1/2
  Product : Product
  Subtract : Sum  Inputs=+-
  Subtract1 : Sum  Inputs=+-
  Tanh : Trigonometry  Operator=tanh
  constant : Constant  Value=4
  time : simulink/Sources/Ramp  slope=1  start=0  InitialOutput=0
  ref : Outport
  wires:
  final/1 -> Subtract/1
  initial/1 -> Add2/1, Subtract/2
  Subtract/1 -> Gain/1
  Gain/1 -> Add2/2, Product/1  "a"
  constant/1 -> Add/1
  step_time/1 -> Add/2
  Add/1 -> Subtract1/2  "x_center"
  time/1 -> Subtract1/1
  Subtract1/1 -> Tanh/1
  Tanh/1 -> Product/2
  Product/1 -> Add1/1
  Add2/1 -> Add1/2  "y_center"
  Add1/1 -> ref/1

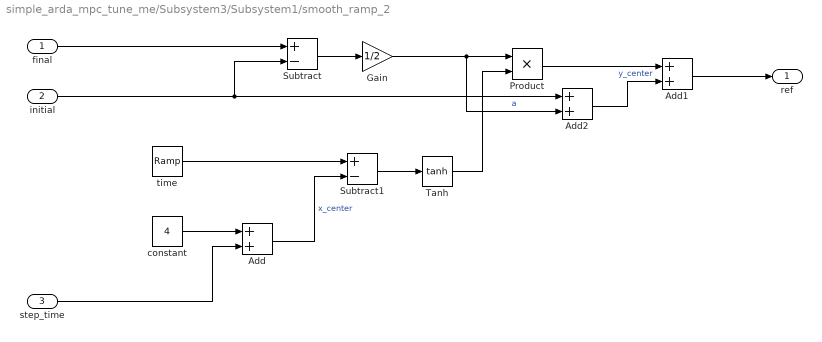
== system simple_arda_mpc_tune_me/Subsystem3/Subsystem1/smooth_ramp_2 ==
  final : Inport
  initial : Inport  Port=2
  step_time : Inport  Port=3
  Add : Sum
  Add1 : Sum
  Add2 : Sum
  Gain : Gain  Gain=1/2
  Product : Product
  Subtract : Sum  Inputs=+-
  Subtract1 : Sum  Inputs=+-
  Tanh : Trigonometry  Operator=tanh
  constant : Constant  Value=4
  time : simulink/Sources/Ramp  slope=1  start=0  InitialOutput=0
  ref : Outport
  wires:
  Add1/1 -> ref/1
  Add2/1 -> Add1/2  "y_center"
  Product/1 -> Add1/1
  Tanh/1 -> Product/2
  Subtract1/1 -> Tanh/1
  time/1 -> Subtract1/1
  Add/1 -> Subtract1/2  "x_center"
  step_time/1 -> Add/2
  constant/1 -> Add/1
  Gain/1 -> Product/1, Add2/2  "a"
  Subtract/1 -> Gain/1
  initial/1 -> Subtract/2, Add2/1
  final/1 -> Subtract/1

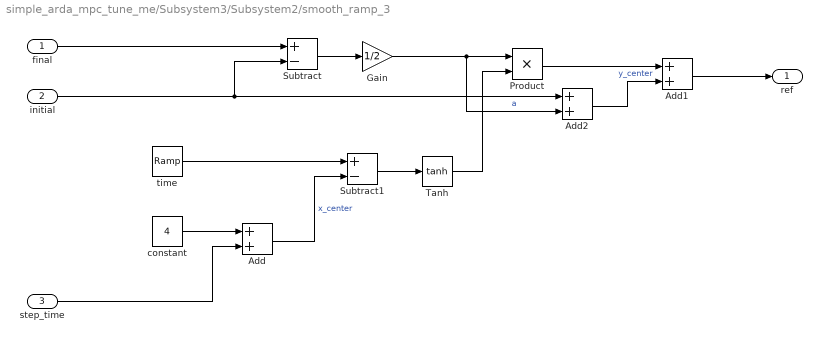
== system simple_arda_mpc_tune_me/Subsystem3/Subsystem2/smooth_ramp_3 ==
  final : Inport
  initial : Inport  Port=2
  step_time : Inport  Port=3
  Add : Sum
  Add1 : Sum
  Add2 : Sum
  Gain : Gain  Gain=1/2
  Product : Product
  Subtract : Sum  Inputs=+-
  Subtract1 : Sum  Inputs=+-
  Tanh : Trigonometry  Operator=tanh
  constant : Constant  Value=4
  time : simulink/Sources/Ramp  slope=1  start=0  InitialOutput=0
  ref : Outport
  wires:
  final/1 -> Subtract/1
  initial/1 -> Add2/1, Subtract/2
  Subtract/1 -> Gain/1
  Gain/1 -> Add2/2, Product/1  "a"
  constant/1 -> Add/1
  step_time/1 -> Add/2
  Add/1 -> Subtract1/2  "x_center"
  time/1 -> Subtract1/1
  Subtract1/1 -> Tanh/1
  Tanh/1 -> Product/2
  Product/1 -> Add1/1
  Add2/1 -> Add1/2  "y_center"
  Add1/1 -> ref/1
